simulink model "phase_lead_control_with_pi_closed_loop_system"  (R2020b)
settings: Solver=VariableStepAuto  StartTime=0.0  StopTime=200  RelTol=1e-3
values from neighbouring files (symbols this model uses):
  COMMANDED_TORQUE_SATURATION = 0.05    [Workshop_MATLAB.m]
  COUPLING_COEFFICIENT = 0.5736    [Workshop_MATLAB.m]
  DISTURBANCE_TORQUE = 0.001    [Workshop_MATLAB.m]
  DISTURBANCE_TORQUE_DELAY = 100    [Workshop_MATLAB.m]
  FLEXIBLE_MODE_DAMPING_RATIO = 0.00495    [Workshop_MATLAB.m]
  FLEXIBLE_MODE_FREQUENCY = 2.6268    [Workshop_MATLAB.m]
  INITIAL_CONDITION_ON_STATE = 0.0001    [Workshop_MATLAB.m]
  MEASUREMENT_DELAY = 0.8    [Workshop_MATLAB.m]
  MEASUREMENT_NOISE_VARIANCE = 10^(-9)    (= 1e-09)    [Workshop_MATLAB.m]
  MODAL_CONTROL_WITH_INTEGRATOR_MAXIMUM_TOLERABLE_POINTING_ERROR = 5 *(2*pi/360)    (= 0.0872664625997)    [Workshop_MATLAB.m]
  phaseLeadPiTransferFunctionDenominator = [phaseLeadPiTimeConstant 0]    [Workshop_MATLAB.m]
  phaseLeadPiTransferFunctionNumerator = [phaseLeadPiTimeConstant 1]    [Workshop_MATLAB.m]
  phaseLeadWithPiControllerTransferFunctionDenominator = phaseLeadOptimizedControllerTransferFunctionDenominator    [Workshop_MATLAB.m]
  phaseLeadWithPiControllerTransferFunctionNumerator = phaseLeadPiInducedAdditionalGain*phaseLeadOptimizedControllerTransferFunctionNumerator    [Workshop_MATLAB.m]
  phaseLeadWithPiFeedForwardGain = dcgain(phaseLeadWithPiControllerTransferFunction)    [Workshop_MATLAB.m]
  REACTION_WHEEL_DYNAMICS_DENOMINATOR = [1 2.400 0.763]    [Workshop_MATLAB.m]
  REACTION_WHEEL_DYNAMICS_NUMERATOR = REACTION_WHEEL_INERTIA*[1.214 0.763 0]    [Workshop_MATLAB.m]
  REACTION_WHEEL_INERTIA = 0.0004    [Workshop_MATLAB.m]
  REACTION_WHEEL_VELOCITY_SATURATION = 2800*2*pi/60    (= 293.215314335)    [Workshop_MATLAB.m]
  SATELLITE_INERTIA = 31.38    [Workshop_MATLAB.m]
  STAR_TRACKER_NOISE_DELAY = 160    [Workshop_MATLAB.m]
settings Model: Creator=WLCG  LastModifiedBy=WLCG

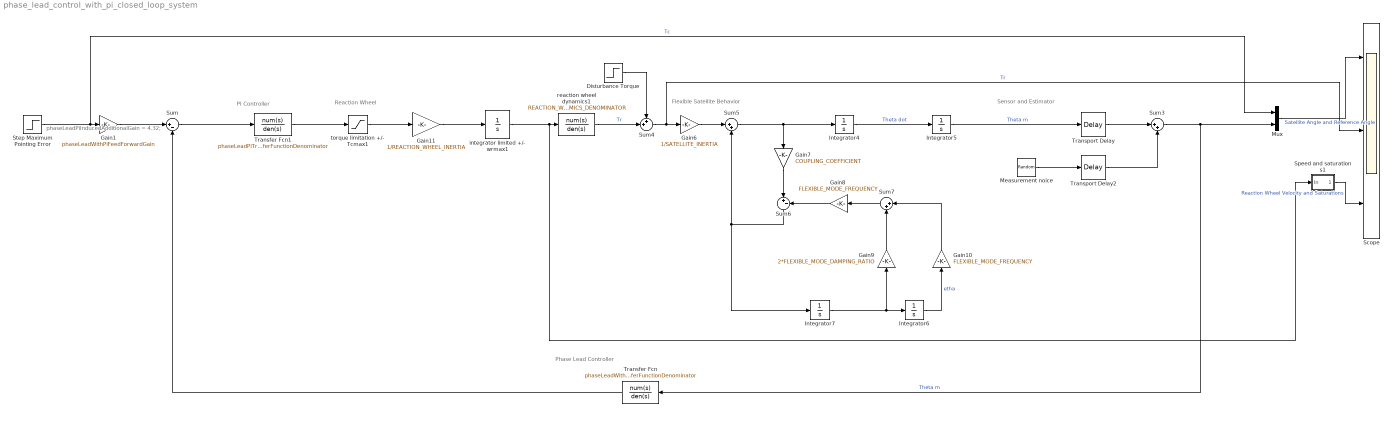
== system phase_lead_control_with_pi_closed_loop_system ==
  note: phaseLeadPiInducedAdditionalGain = 4.32;
  note: PI Controller
  note: Phase Lead Controller
  note: Flexible Satellite Behavior
  note: Reaction Wheel
  note: Sensor and Estimator
  Disturbance Torque : Step  Time=DISTURBANCE_TORQUE_DELAY  After=DISTURBANCE_TORQUE  SampleTime=0
  Gain1 : Gain  Gain=phaseLeadWithPiFeedForwardGain
  Gain10 : Gain  Gain=FLEXIBLE_MODE_FREQUENCY
  Gain11 : Gain  Gain=1/REACTION_WHEEL_INERTIA
  Gain6 : Gain  Gain=1/SATELLITE_INERTIA
  Gain7 : Gain  Gain=COUPLING_COEFFICIENT
  Gain8 : Gain  Gain=FLEXIBLE_MODE_FREQUENCY
  Gain9 : Gain  Gain=2*FLEXIBLE_MODE_DAMPING_RATIO
  Integrator4 : Integrator
  Integrator5 : Integrator
  Integrator6 : Integrator  InitialCondition=INITIAL_CONDITION_ON_STATE
  Integrator7 : Integrator
  Measurement noice : RandomNumber  Variance=MEASUREMENT_NOISE_VARIANCE  SampleTime=0.01
  Mux : Mux  Inputs=2
  Scope : Scope  NumInputPorts=3
  Speed and saturations1 : Subsystem
  Step Maximum Pointing Error : Step  Time=0  After=MODAL_CONTROL_WITH_INTEGRATOR_MAXIMUM_TOLERABLE_POINTING_ERROR  SampleTime=0
  Sum : Sum  Inputs=|+-
  Sum3 : Sum  Inputs=|++
  Sum4 : Sum  Inputs=++|
  Sum5 : Sum  Inputs=|++
  Sum6 : Sum  Inputs=|+-
  Sum7 : Sum  Inputs=|++
  Transfer Fcn : TransferFcn  Numerator=phaseLeadWithPiControllerTransferFunctionNumerator  Denominator=phaseLeadWithPiControllerTransferFunctionDenominator
  Transfer Fcn1 : TransferFcn  Numerator=phaseLeadPiTransferFunctionNumerator  Denominator=phaseLeadPiTransferFunctionDenominator
  Transport Delay : TransportDelay  DelayTime=MEASUREMENT_DELAY
  Transport Delay2 : TransportDelay  DelayTime=STAR_TRACKER_NOISE_DELAY
  integrator limited +/- wrmax1 : Integrator  LimitOutput=on  UpperSaturationLimit=REACTION_WHEEL_VELOCITY_SATURATION  LowerSaturationLimit=-REACTION_WHEEL_VELOCITY_SATURATION
  reaction wheel dynamics1 : TransferFcn  Numerator=REACTION_WHEEL_DYNAMICS_NUMERATOR  Denominator=REACTION_WHEEL_DYNAMICS_DENOMINATOR
  torque limitation +/- Tcmax1 : Saturate  UpperLimit=COMMANDED_TORQUE_SATURATION  LowerLimit=-COMMANDED_TORQUE_SATURATION
  wires:
  Gain7/1 -> Sum6/1
  Gain9/1 -> Sum7/2
  Sum7/1 -> Gain8/1
  Gain10/1 -> Sum7/1
  Gain8/1 -> Sum6/2
  Integrator4/1 -> Integrator5/1  "Theta dot"
  torque limitation +/- Tcmax1/1 -> Gain11/1
  Gain6/1 -> Sum5/1
  Gain11/1 -> integrator limited +/- wrmax1/1
  Sum5/1 -> Gain7/1, Integrator4/1
  Integrator6/1 -> Gain10/1  "etha"
  Integrator7/1 -> Integrator6/1, Gain9/1
  integrator limited +/- wrmax1/1 -> Speed and saturations1/1(In), reaction wheel dynamics1/1
  Sum6/1 -> Sum5/2, Integrator7/1
  Gain1/1 -> Sum/1
  Transfer Fcn/1 -> Sum/2
  Disturbance Torque/1 -> Sum4/1
  reaction wheel dynamics1/1 -> Sum4/2  "Tr"
  Sum4/1 -> Scope/2, Gain6/1  "Tr"
  Transport Delay2/1 -> Sum3/2
  Transport Delay/1 -> Sum3/1
  Measurement noice/1 -> Transport Delay2/1
  Sum3/1 -> Transfer Fcn/1, Mux/2  "Theta m"
  Integrator5/1 -> Transport Delay/1  "Theta m"
  Mux/1 -> Scope/1  "Satellite Angle and Reference Angle"
  Step Maximum Pointing Error/1 -> Mux/1, Gain1/1  "Tc"
  Sum/1 -> Transfer Fcn1/1
  Transfer Fcn1/1 -> torque limitation +/- Tcmax1/1
  Speed and saturations1/1(Mux) -> Scope/3  "Reaction Wheel Velocity and Saturations"

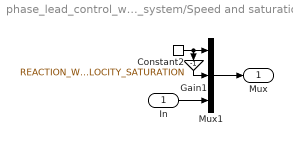
== system phase_lead_control_with_pi_closed_loop_system/Speed and saturations1 ==
  In : Inport
  Constant2 : Constant  Value=REACTION_WHEEL_VELOCITY_SATURATION
  Gain1 : Gain  Gain=-1
  Mux1 : Mux  Inputs=3
  Mux : Outport
  wires:
  Gain1/1 -> Mux1/2
  In/1 -> Mux1/3
  Mux1/1 -> Mux/1
  Constant2/1 -> Gain1/1, Mux1/1
